simulink model "example3sim"  (Simulink 8.8)
settings: Solver=ode45  StartTime=0.0  StopTime=Tstop  RelTol=1e-3  EnableMultiTasking=on
values from neighbouring files (symbols this model uses):
  C1 = lincon(model,'track',cost,interval,limits)    [example1.m]    (also in example3.m; timevarying1.m = lincon(themodel,'track',cost,interval,limits); varbounds.m = kalmdesign(C1,Qn,Rn,ymeasured))
libraries: cstblocks x1, hyblib x1
settings Model: SuppressorTable=22 serialization::archive 11 0 3 0 0 0 0 0  Creator=bemporad  LastModifiedBy=bemporad  ExtModeTrigMode=oneshot  ExtModeArmWhenConnect=off
settings DataIOCC: LimitDataPoints=off  SignalLoggingName=sigsOut
settings OptimizationCC: BooleanDataType=off  LifeSpan=auto
settings DebuggingCC: SaveWithParameterizedLinksMsg=none  SignalResolutionControl=TryResolveAllWithWarning  MultiTaskDSMMsg=warning  MultiTaskCondExecSysMsg=none  FcnCallInpInsideContextMsg=error  StateNameClashWarn=none  SFUnexpectedBacktrackingDiag=error  SFNoUnconditionalDefaultTransitionDiag=error  SFExecutionAtInitializationDiag=warning
settings HardwareCC: TargetUnknown=on
settings GRTTargetCC: GeneratePreprocessorConditionals=Use local settings

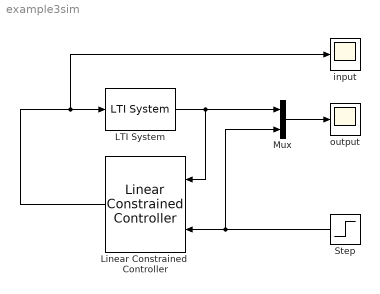
== system example3sim ==
  LTI System : cstblocks/LTI System  sys=tf(1,[1 .4 1])  IC=[]
  Linear Constrained  Controller : hyblib/Linear Constrained  Controller  C=C1  xhat0=[]  u1=0
  Mux : Mux  Inputs=2
  Step : Step  Time=0  Before=1  SampleTime=0
  input : Scope
  output : Scope
  wires:
  LTI System/1 -> Mux/1, Linear Constrained  Controller/1
  Mux/1 -> output/1
  Linear Constrained  Controller/1 -> input/1, LTI System/1
  Step/1 -> Linear Constrained  Controller/2, Mux/2
